simulink model "untitled2"  (R2023b)
settings: Solver=VariableStepAuto  StartTime=0.0  StopTime=100  RelTol=1e-3
undefined symbols (not defined in the file): magnitude
libraries: dspfdesign x1
settings Model: Creator=mrabd  LastModifiedBy=mrabd

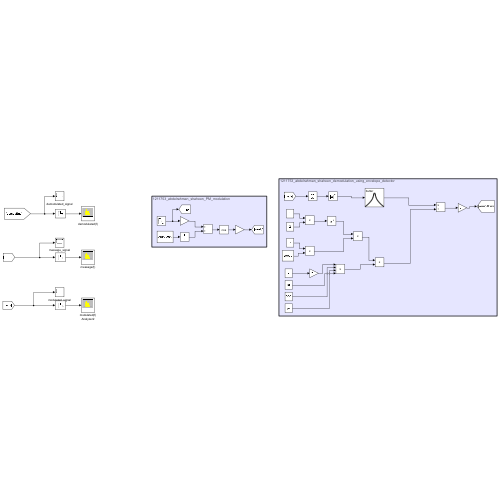
[thumbnail: Simulink's stored preview of the top-level diagram]
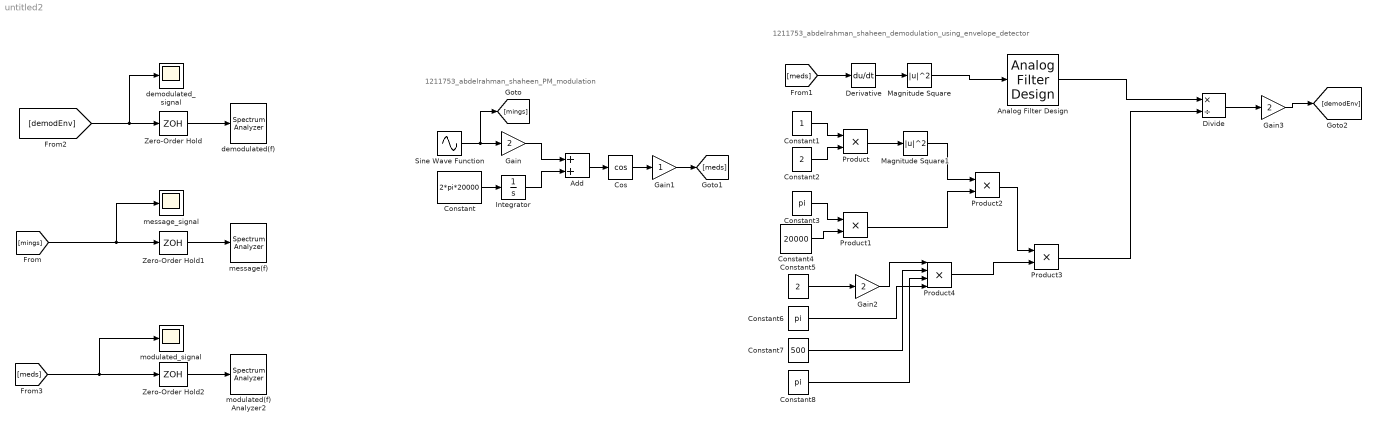
== system untitled2 ==
  note: 1211753_abdelrahman_shaheen_demodulation_using_envelope_detector
  note: 1211753_abdelrahman_shaheen_PM_modulation
  Add : Sum
  Analog Filter Design : dspfdesign/Analog Filter Design  method=Butterworth  filttype=Bandpass  N=4  Wlo=450  Whi=550  Rp=2  Rs=40
  Constant : Constant  Value=2*pi*20000
  Constant1 : Constant
  Constant2 : Constant  Value=2
  Constant3 : Constant  Value=pi
  Constant4 : Constant  Value=20000
  Constant5 : Constant  Value=2
  Constant6 : Constant  Value=pi
  Constant7 : Constant  Value=500
  Constant8 : Constant  Value=pi
  Cos : Trigonometry  Operator=cos
  Derivative : Derivative
  Divide : Product  Inputs=*/
  Gain : Gain  Gain=2
  Gain1 : Gain
  Gain2 : Gain  Gain=2
  Gain3 : Gain  Gain=2
  Integrator : Integrator
  Magnitude Square : Math  Operator=magnitude^2  SignedPower=on  RndMeth=Zero
  Magnitude Square1 : Math  Operator=magnitude^2  SignedPower=on  RndMeth=Zero
  Product{,1..3} (4 alike) : Product
  Product4 : Product  Inputs=4
  Sine Wave Function : Sin  Amplitude=pi  Frequency=500  SampleTime=0
  Zero-Order Hold : ZeroOrderHold  SampleTime=-1
  Zero-Order Hold1 : ZeroOrderHold  SampleTime=-1
  Zero-Order Hold2 : ZeroOrderHold  SampleTime=-1
  demodulated(f) : SpectrumAnalyzer  WindowPosition=[368.000000,182.000000,800.000000,500.000000,]  ScopeFrameLocation=window  SampleRateSource=Property  SampleRate=44.1e3  PlotAsTwoSidedSpectrum=off  FrequencyScale=Log  FrequencySpan=Start and stop frequencies  StartFrequency=20  StopFrequency=20e3  YLimits=[-133.55827494,-38.22367633]
  demodulated_signal : Scope
  message(f) : SpectrumAnalyzer  WindowPosition=[368.000000,182.000000,800.000000,500.000000,]  ScopeFrameLocation=window  SampleRateSource=Property  SampleRate=44.1e3  PlotAsTwoSidedSpectrum=off  FrequencyScale=Log  FrequencySpan=Start and stop frequencies  StartFrequency=20  StopFrequency=20e3  YLimits=[-57.49782481,43.02326432]
  message_signal : Scope
  modulated(f) Analyzer2 : SpectrumAnalyzer  WindowPosition=[368.000000,182.000000,800.000000,500.000000,]  ScopeFrameLocation=window  SampleRateSource=Property  SampleRate=44.1e3  PlotAsTwoSidedSpectrum=off  FrequencyScale=Log  FrequencySpan=Start and stop frequencies  StartFrequency=20  StopFrequency=20e3  YLimits=[-61.73421248,29.43500858]
  modulated_signal : Scope
  wires:
  Gain/1 -> Add/1
  Gain1/1 -> [meds]
  Add/1 -> Cos/1
  Sine Wave Function/1 -> [mings], Gain/1
  Cos/1 -> Gain1/1
  Integrator/1 -> Add/2
  Constant/1 -> Integrator/1
  [meds] -> Derivative/1
  Constant8/1 -> Product4/3
  Constant7/1 -> Product4/2
  Derivative/1 -> Magnitude Square/1
  Product2/1 -> Product3/1
  Product4/1 -> Product3/2
  Gain3/1 -> [demodEnv]
  Gain2/1 -> Product4/1
  Divide/1 -> Gain3/1
  Product/1 -> Magnitude Square1/1
  Product3/1 -> Divide/2
  Product1/1 -> Product2/2
  Constant6/1 -> Product4/4
  Constant3/1 -> Product1/1
  Constant2/1 -> Product/2
  Analog Filter Design/1 -> Divide/1
  Constant4/1 -> Product1/2
  Magnitude Square/1 -> Analog Filter Design/1
  Magnitude Square1/1 -> Product2/1
  Constant5/1 -> Gain2/1
  Constant1/1 -> Product/1
  [demodEnv] -> Zero-Order Hold/1, demodulated_signal/1
  [mings] -> message_signal/1, Zero-Order Hold1/1
  [meds] -> modulated_signal/1, Zero-Order Hold2/1
  Zero-Order Hold/1 -> demodulated(f)/1
  Zero-Order Hold1/1 -> message(f)/1
  Zero-Order Hold2/1 -> modulated(f) Analyzer2/1
